simulink model "Lecture15_DigitalLSF"  (R2020b)
settings: Solver=VariableStepAuto  StartTime=0.0  StopTime=10.0  RelTol=1e-3
values from neighbouring files (symbols this model uses):
  Cd = C    [Assignment4.m]    (also in Lecture15_DigitalLSF.m)
  K = 1.5    [Assignment1.m]    (also in Assignment4.m = acker(A_mark, B_mark, s_p); Lecture14_LSF.m = [1.25, 1]; Lecture15_DigitalLSF.m = acker(Ad, Bd, [z_p, z_p]); Lecture16_LSFIntegrator.m = acker(A_mark, B_mark, [s_p, s_p, s_p]))
  T = 1/((20*wc)/(2*pi))    (= 0.0010471975512)    [Assignment1.m]    (also in Assignment3.m = [1/(2.5*bw) 1/(10*bw) 1/(25*bw)]; Lecture15_DigitalLSF.m = 1 / ((25 * bandwidth(tf([10], [2 2 1])))); Lecture4_DiscretePID.m = 0.1)
undefined symbols (not defined in the file or in its folder): Ad, Bd
settings Model: Creator=sebastian  LastModifiedBy=sebastian

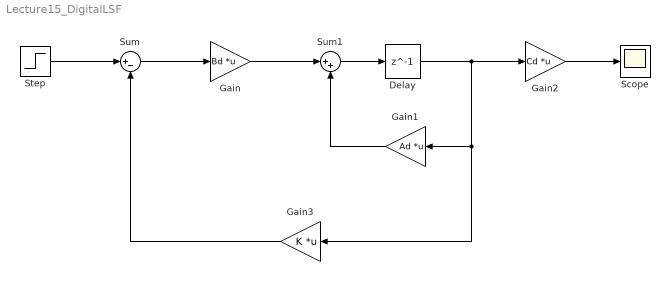
== system Lecture15_DigitalLSF ==
  Delay : Delay  DelayLength=1  InitialCondition=0  SampleTime=T
  Gain : Gain  Gain=Bd  Multiplication=Matrix(K*u)
  Gain1 : Gain  Gain=Ad  Multiplication=Matrix(K*u)
  Gain2 : Gain  Gain=Cd  Multiplication=Matrix(K*u)
  Gain3 : Gain  Gain=K  Multiplication=Matrix(K*u)
  Scope : Scope
  Step : Step  SampleTime=0
  Sum : Sum  Inputs=|+-
  Sum1 : Sum  Inputs=|++
  wires:
  Step/1 -> Sum/1
  Sum/1 -> Gain/1
  Gain/1 -> Sum1/1
  Sum1/1 -> Delay/1
  Delay/1 -> Gain3/1, Gain1/1, Gain2/1
  Gain1/1 -> Sum1/2
  Gain2/1 -> Scope/1
  Gain3/1 -> Sum/2
